simulink model "lookupTableDynamic_TestGen3"  (R2017b)
settings: Solver=FixedStepDiscrete  StartTime=0.0  StopTime=10.0  RelTol=1e-3
libraries: simulink x1
settings Model: Creator=ktrinh  LastModifiedBy=ktrinh
settings DebuggingCC: ParameterOverflowMsg=none

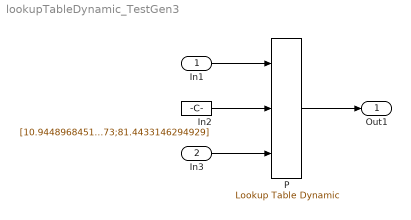
== system lookupTableDynamic_TestGen3 ==
  In1 : Inport  OutMin=8.9449  OutMax=83  OutDataTypeStr=int8  PortDimensions=[2,3]
  In3 : Inport  Port=2  PortDimensions=5
  In2 : Constant  Value=[10.9448968451437;47.926132668027;53.2503685843485;68.8685424780073;81.4433146294929]  OutDataTypeStr=int8
  P : simulink/Lookup Tables/Lookup Table Dynamic  LookUpMeth=Interpolation-Extrapolation  OutDataType=fixdt('int8')  OutScaling=[]  OutputDataTypeScalingMode=Specify via dialog  OutDataTypeStr=int8  RndMeth=Nearest  DoSatur=on
      settings: SourceProductName=Simulink
  Out1 : Outport
  wires:
  In1/1 -> P/1
  In2/1 -> P/2
  In3/1 -> P/3
  P/1 -> Out1/1
